simulink model "groundhookidealMRcom"  (R2016a)
settings: Solver=VariableStepAuto  StartTime=0.0  StopTime=10.0  RelTol=1e-3
undefined symbols (not defined in the file): b1, k1, k2, m1, m2
settings Model: Creator=mm395  LastModifiedBy=mm395

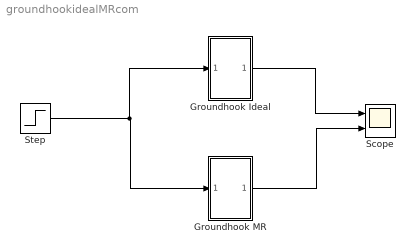
== system groundhookidealMRcom ==
  Groundhook Ideal : Subsystem
  Groundhook MR : Subsystem
  Scope : Scope  NumInputPorts=2
  Step : Step
  wires:
  Step/1 -> Groundhook Ideal/1(In1), Groundhook MR/1(In2)
  Groundhook MR/1(Out2) -> Scope/2
  Groundhook Ideal/1(Out1) -> Scope/1

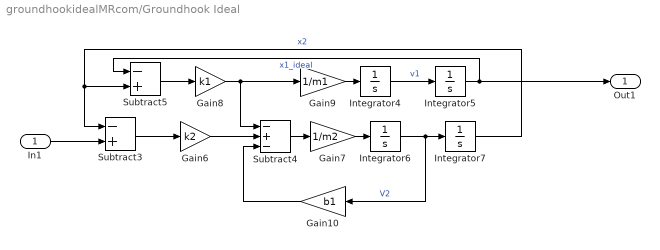
== system groundhookidealMRcom/Groundhook Ideal ==
  In1 : Inport
  Gain10 : Gain  Gain=b1
  Gain6 : Gain  Gain=k2
  Gain7 : Gain  Gain=1/m2
  Gain8 : Gain  Gain=k1
  Gain9 : Gain  Gain=1/m1
  Integrator{4..7} (4 alike) : Integrator
  Subtract3 : Sum  Inputs=-+
  Subtract4 : Sum  Inputs=-+-
  Subtract5 : Sum  Inputs=-+
  Out1 : Outport
  wires:
  Gain9/1 -> Integrator4/1
  Gain7/1 -> Integrator6/1
  Integrator6/1 -> Integrator7/1, Gain10/1  "V2"
  Integrator4/1 -> Integrator5/1  "v1"
  Integrator5/1 -> Subtract5/1, Out1/1  "x1_ideal"
  Gain10/1 -> Subtract4/3
  Subtract5/1 -> Gain8/1
  In1/1 -> Subtract3/2
  Subtract4/1 -> Gain7/1
  Gain8/1 -> Gain9/1, Subtract4/1
  Integrator7/1 -> Subtract3/1, Subtract5/2  "x2"
  Gain6/1 -> Subtract4/2
  Subtract3/1 -> Gain6/1

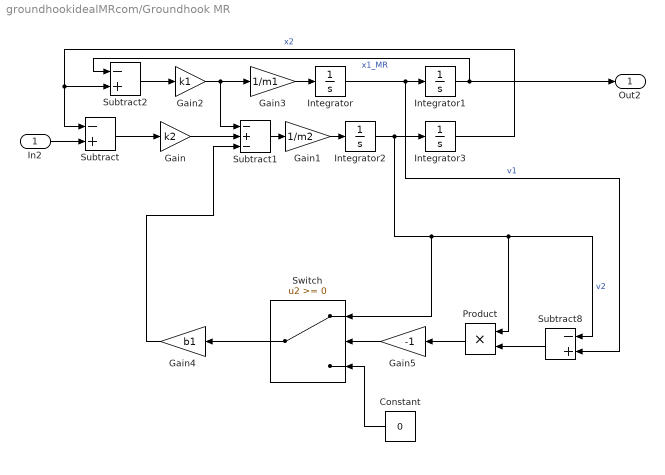
== system groundhookidealMRcom/Groundhook MR ==
  In2 : Inport
  Constant : Constant  Value=0
  Gain : Gain  Gain=k2
  Gain1 : Gain  Gain=1/m2
  Gain2 : Gain  Gain=k1
  Gain3 : Gain  Gain=1/m1
  Gain4 : Gain  Gain=b1
  Gain5 : Gain  Gain=-1
  Integrator{,1..3} (4 alike) : Integrator
  Product : Product
  Subtract : Sum  Inputs=-+
  Subtract1 : Sum  Inputs=-+-
  Subtract2 : Sum  Inputs=-+
  Subtract8 : Sum  Inputs=-+
  Switch : Switch  ZeroCross=off
  Out2 : Outport
  wires:
  Switch/1 -> Gain4/1
  Integrator3/1 -> Subtract/1, Subtract2/2  "x2"
  Gain/1 -> Subtract1/2
  Subtract/1 -> Gain/1
  Subtract1/1 -> Gain1/1
  In2/1 -> Subtract/2
  Gain2/1 -> Gain3/1, Subtract1/1
  Subtract2/1 -> Gain2/1
  Gain3/1 -> Integrator/1
  Integrator/1 -> Integrator1/1, Subtract8/2  "v1"
  Gain1/1 -> Integrator2/1
  Gain4/1 -> Subtract1/3
  Integrator1/1 -> Out2/1, Subtract2/1  "x1_MR"
  Integrator2/1 -> Integrator3/1, Switch/1, Product/1, Subtract8/1  "v2"
  Product/1 -> Gain5/1
  Subtract8/1 -> Product/2
  Gain5/1 -> Switch/2
  Constant/1 -> Switch/3
